simulink model "week2_3"  (R2020b)
settings: Solver=VariableStepAuto  StartTime=0.0  StopTime=10  RelTol=1e-3
model workspace (MAT data in the model file):
  Ki = Simulink.Parameter
  Ki.Value = 40
  Ki.DataType = 'auto'
  Ki.Dimensions = [1 1]
  Kp = Simulink.Parameter
  Kp.Value = 800
  Kp.DataType = 'auto'
  Kp.Dimensions = [1 1]
  b = Simulink.Parameter
  b.Value = 50
  b.DataType = 'auto'
  b.Dimensions = [1 1]
  m = Simulink.Parameter
  m.Value = 1000
  m.DataType = 'auto'
  m.Dimensions = [1 1]
  u = Simulink.Parameter
  u.Value = 500
  u.DataType = 'auto'
  u.Dimensions = [1 1]
values from neighbouring files (symbols this model uses):
  b = 500    [varset.m]
  m = 1000    [varset.m]
settings Model: Creator=lalit  LastModifiedBy=lalit

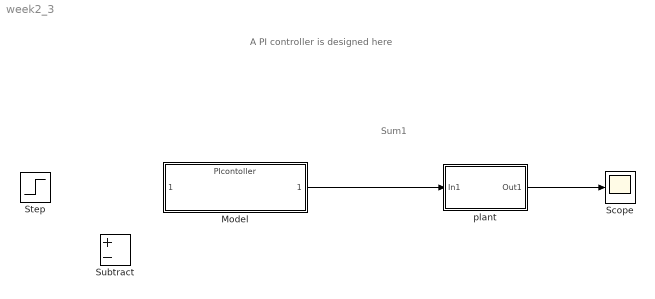
== system week2_3 ==
  note: A PI controller is designed here
  note: Sum1
  Model : ModelReference  ModelNameDialog=PIcontoller.slx  SimulationMode=Normal  ModelReferenceVersion=1.18
  Scope : Scope
  Step : Step  SampleTime=0
  Subtract : Sum  Inputs=+-
  "plant " : Subsystem
  wires:
  "plant "/1(Out1) -> Scope/1
  Model/1 -> "plant "/1(In1)

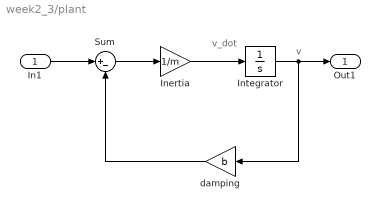
== system week2_3/plant  ==
  note: v_dot
  note: v
  In1 : Inport
  Inertia : Gain  Gain=1/m
  Integrator : Integrator
  Sum : Sum  Inputs=|+-
  damping : Gain  Gain=b
  Out1 : Outport
  wires:
  In1/1 -> Sum/1
  Sum/1 -> Inertia/1
  Inertia/1 -> Integrator/1
  damping/1 -> Sum/2
  Integrator/1 -> Out1/1, damping/1
